simulink model "bldc_foc"  (Simulink 8.0)
settings: Solver=ode45  StartTime=0.0  StopTime=5  MaxStep=1e-4  RelTol=1e-3
libraries: BLDC x1
settings Model: Creator=Rodrigo  LastModifiedBy=h3now
settings DataIOCC: SignalLoggingSaveFormat=ModelDataLogs
settings DebuggingCC: FcnCallInpInsideContextMsg=EnableAllAsWarning
settings GRTTargetCC: CombineOutputUpdateFcns=off  GRTInterface=on
settings ConfigurationSet: Description=SimMechanics 2G

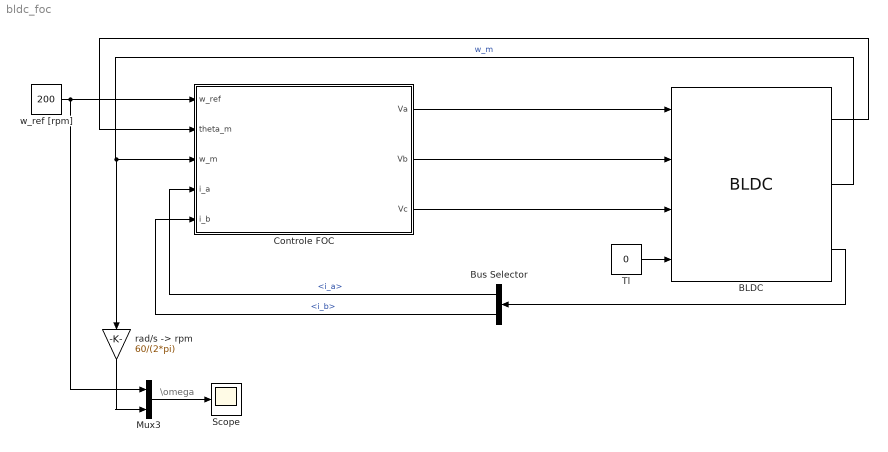
== system bldc_foc ==
  note: \omega
  BLDC : BLDC/BLDC  J=3.84e-7 + 1e-4  R=23.9/2  L=2.35e-3/2  P=8  Kt=11.3e-3  Ke=11.3e-3  Kd=0  default_fcem=on  fcem_a=fcem_a  fcem_b=fcem_b  fcem_c=fcem_c
  Bus Selector : BusSelector  OutputSignals=Correntes.i_a,Correntes.i_b
  Controle FOC : Subsystem
  Mux3 : Mux  Inputs=2
  Scope : Scope
      settings: TimeRange=10  YMin=20  YMax=200  Decimation=10
  Tl : Constant  Value=0
  "rad/s -> rpm" : Gain  Gain=60/(2*pi)
  w_ref [rpm] : Constant  Value=200
  wires:
  BLDC/3 -> Bus Selector/1
  Tl/1 -> BLDC/4
  Mux3/1 -> Scope/1
  BLDC/1 -> Controle FOC/2(theta_m)
  BLDC/2 -> "rad/s -> rpm"/1, Controle FOC/3(w_m)  "w_m"
  Controle FOC/1(Va) -> BLDC/1
  Controle FOC/2(Vb) -> BLDC/2
  Controle FOC/3(Vc) -> BLDC/3
  w_ref [rpm]/1 -> Mux3/1, Controle FOC/1(w_ref)
  "rad/s -> rpm"/1 -> Mux3/2
  Bus Selector/1 -> Controle FOC/4(i_a)  "<i_a>"
  Bus Selector/2 -> Controle FOC/5(i_b)  "<i_b>"

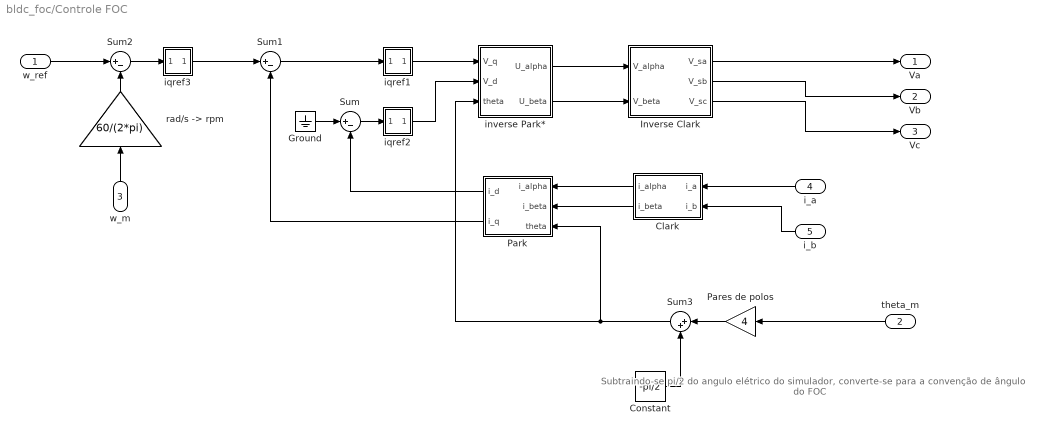
== system bldc_foc/Controle FOC ==
  note: Subtraindo-se pi/2 do angulo elétrico do simulador,
      | converte-se para a convenção de ângulo do FOC
  w_ref : Inport
  theta_m : Inport  Port=2
  w_m : Inport  Port=3
  i_a : Inport  Port=4
  i_b : Inport  Port=5
  Clark : Subsystem
  Constant : Constant  Value=-pi/2
  Ground : Ground
  Inverse Clark : Subsystem
  Pares de polos : Gain  Gain=4
  Park : Subsystem
  Sum : Sum  Inputs=|+-
  Sum1 : Sum  Inputs=|+-
  Sum2 : Sum  Inputs=|+-
  Sum3 : Sum  Inputs=|++
  inverse Park* : Subsystem
  iqref1 : Subsystem  mask(PI Controller){I=0.5, P=1, sat=[-500, 500]}
      mask prompts: I "Integral"; P "Proportional:"; sat "Minimum and maximum outputs:"
      mask init:
      | min=sat(1);max=sat(2);
      mask Display: disp('PI')
  iqref2 : Subsystem  mask(PI Controller){I=5, P=10, sat=[-500, 500]}
      mask prompts: I "Integral"; P "Proportional:"; sat "Minimum and maximum outputs:"
      mask init:
      | min=sat(1);max=sat(2);
      mask Display: disp('PI')
  iqref3 : Subsystem  mask(PI Controller){I=0.1, P=0.1, sat=[-500, 500]}
      mask prompts: I "Integral"; P "Proportional:"; sat "Minimum and maximum outputs:"
      mask init:
      | min=sat(1);max=sat(2);
      mask Display: disp('PI')
  "rad/s -> rpm" : Gain  Gain=60/(2*pi)
  Va : Outport
  Vb : Outport  Port=2
  Vc : Outport  Port=3
  wires:
  inverse Park*/2(U_beta) -> Inverse Clark/2(V_beta)
  inverse Park*/1(U_alpha) -> Inverse Clark/1(V_alpha)
  Clark/1(i_alpha) -> Park/1(i_alpha)
  Clark/2(i_beta) -> Park/2(i_beta)
  Sum/1 -> iqref2/1(In_1)
  Park/1(i_d) -> Sum/2
  Ground/1 -> Sum/1
  w_m/1 -> "rad/s -> rpm"/1
  iqref2/1(Out_1) -> inverse Park*/2(V_d)
  Sum3/1 -> Park/3(theta), inverse Park*/3(theta)
  Park/2(i_q) -> Sum1/2
  "rad/s -> rpm"/1 -> Sum2/2
  iqref1/1(Out_1) -> inverse Park*/1(V_q)
  i_a/1 -> Clark/1(i_a)
  Inverse Clark/3(V_sc) -> Vc/1
  Inverse Clark/1(V_sa) -> Va/1
  iqref3/1(Out_1) -> Sum1/1
  Sum2/1 -> iqref3/1(In_1)
  Inverse Clark/2(V_sb) -> Vb/1
  Sum1/1 -> iqref1/1(In_1)
  i_b/1 -> Clark/2(i_b)
  w_ref/1 -> Sum2/1
  Constant/1 -> Sum3/2
  Pares de polos/1 -> Sum3/1
  theta_m/1 -> Pares de polos/1

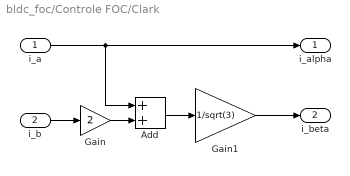
== system bldc_foc/Controle FOC/Clark ==
  i_a : Inport
  i_b : Inport  Port=2
  Add : Sum
  Gain : Gain  Gain=2
  Gain1 : Gain  Gain=1/sqrt(3)
  i_alpha : Outport
  i_beta : Outport  Port=2
  wires:
  i_a/1 -> i_alpha/1, Add/1
  i_b/1 -> Gain/1
  Gain/1 -> Add/2
  Add/1 -> Gain1/1
  Gain1/1 -> i_beta/1

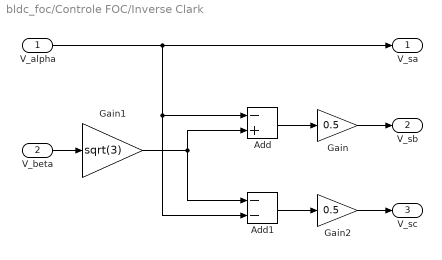
== system bldc_foc/Controle FOC/Inverse Clark ==
  V_alpha : Inport
  V_beta : Inport  Port=2
  Add : Sum  Inputs=-+
  Add1 : Sum  Inputs=--
  Gain : Gain  Gain=0.5
  Gain1 : Gain  Gain=sqrt(3)
  Gain2 : Gain  Gain=0.5
  V_sa : Outport
  V_sb : Outport  Port=2
  V_sc : Outport  Port=3
  wires:
  V_alpha/1 -> Add/1, Add1/2, V_sa/1
  Add/1 -> Gain/1
  Gain/1 -> V_sb/1
  Add1/1 -> Gain2/1
  Gain2/1 -> V_sc/1
  V_beta/1 -> Gain1/1
  Gain1/1 -> Add/2, Add1/1

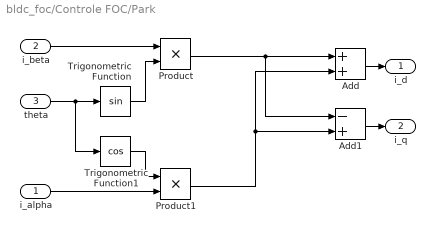
== system bldc_foc/Controle FOC/Park ==
  i_alpha : Inport
  i_beta : Inport  Port=2
  theta : Inport  Port=3
  Add : Sum
  Add1 : Sum  Inputs=-+
  Product : Product  RndMeth=Zero
  Product1 : Product  RndMeth=Zero
  Trigonometric Function : Trigonometry  OutputSignalType=real
  Trigonometric Function1 : Trigonometry  Operator=cos  OutputSignalType=real
  i_d : Outport
  i_q : Outport  Port=2
  wires:
  theta/1 -> Trigonometric Function/1, Trigonometric Function1/1
  i_beta/1 -> Product/1
  Trigonometric Function/1 -> Product/2
  Add/1 -> i_d/1
  Trigonometric Function1/1 -> Product1/1
  i_alpha/1 -> Product1/2
  Product/1 -> Add/1, Add1/1
  Product1/1 -> Add/2, Add1/2
  Add1/1 -> i_q/1

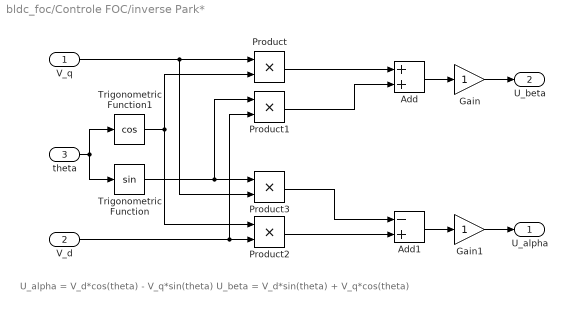
== system bldc_foc/Controle FOC/inverse Park* ==
  note: U_alpha = V_d*cos(theta) - V_q*sin(theta)
      | U_beta = V_d*sin(theta) + V_q*cos(theta)
  V_q : Inport
  V_d : Inport  Port=2
  theta : Inport  Port=3
  Add : Sum
  Add1 : Sum  Inputs=-+
  Gain : Gain
  Gain1 : Gain
  Product{,1..3} (4 alike) : Product  RndMeth=Zero
  Trigonometric Function : Trigonometry  OutputSignalType=real
  Trigonometric Function1 : Trigonometry  Operator=cos  OutputSignalType=real
  U_alpha : Outport
  U_beta : Outport  Port=2
  wires:
  theta/1 -> Trigonometric Function1/1, Trigonometric Function/1
  V_q/1 -> Product/1, Product3/2
  Trigonometric Function1/1 -> Product/2, Product2/1
  V_d/1 -> Product1/2, Product2/2
  Trigonometric Function/1 -> Product1/1, Product3/1
  Product/1 -> Add/1
  Product1/1 -> Add/2
  Product2/1 -> Add1/2
  Product3/1 -> Add1/1
  Add/1 -> Gain/1
  Gain/1 -> U_beta/1
  Add1/1 -> Gain1/1
  Gain1/1 -> U_alpha/1

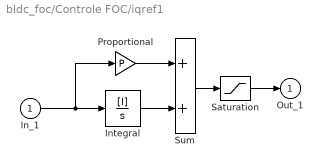
== system bldc_foc/Controle FOC/iqref1 ==
  In_1 : Inport
  Integral : TransferFcn  Numerator=[I]  Denominator=[1 0]
  Proportional : Gain  Gain=P  SaturateOnIntegerOverflow=on  OutDataTypeStr=Inherit: Same as input  ParamDataTypeStr=Inherit: Same as input
  Saturation : Saturate  UpperLimit=max  LowerLimit=min
  Sum : Sum  SaturateOnIntegerOverflow=on  InputSameDT=on  OutDataTypeStr=Inherit: Same as first input
  Out_1 : Outport  InitialOutput=0
  wires:
  Saturation/1 -> Out_1/1
  Sum/1 -> Saturation/1
  Proportional/1 -> Sum/1
  In_1/1 -> Proportional/1, Integral/1
  Integral/1 -> Sum/2

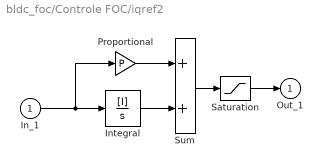
== system bldc_foc/Controle FOC/iqref2 ==
  In_1 : Inport
  Integral : TransferFcn  Numerator=[I]  Denominator=[1 0]
  Proportional : Gain  Gain=P  SaturateOnIntegerOverflow=on  OutDataTypeStr=Inherit: Same as input  ParamDataTypeStr=Inherit: Same as input
  Saturation : Saturate  UpperLimit=max  LowerLimit=min
  Sum : Sum  SaturateOnIntegerOverflow=on  InputSameDT=on  OutDataTypeStr=Inherit: Same as first input
  Out_1 : Outport  InitialOutput=0
  wires:
  Saturation/1 -> Out_1/1
  Sum/1 -> Saturation/1
  Proportional/1 -> Sum/1
  In_1/1 -> Proportional/1, Integral/1
  Integral/1 -> Sum/2

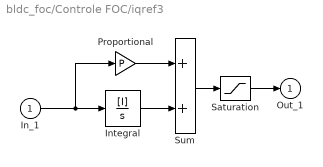
== system bldc_foc/Controle FOC/iqref3 ==
  In_1 : Inport
  Integral : TransferFcn  Numerator=[I]  Denominator=[1 0]
  Proportional : Gain  Gain=P  SaturateOnIntegerOverflow=on  OutDataTypeStr=Inherit: Same as input  ParamDataTypeStr=Inherit: Same as input
  Saturation : Saturate  UpperLimit=max  LowerLimit=min
  Sum : Sum  SaturateOnIntegerOverflow=on  InputSameDT=on  OutDataTypeStr=Inherit: Same as first input
  Out_1 : Outport  InitialOutput=0
  wires:
  Saturation/1 -> Out_1/1
  Sum/1 -> Saturation/1
  Proportional/1 -> Sum/1
  In_1/1 -> Integral/1, Proportional/1
  Integral/1 -> Sum/2
